simulink model "pidcontrol_withmotor"  (Simulink 7.1)
settings: Solver=ode45  StartTime=0.0  StopTime=10  RelTol=1e-3
values from neighbouring files (symbols this model uses):
  f0 = 7.847    [pid_parameters.m]
  f1 = -25.831    [pid_parameters.m]
  g = 9.81    [pid_parameters.m]
  I = 0.00017701    [pid_parameters.m]
  Kd = 0.06*100    (= 6)    [pid_parameters.m]
  Ki = 0.028*100    (= 2.8)    [pid_parameters.m]
  Kp = 0.037*100    (= 3.7)    [pid_parameters.m]
  l = 0.14875    [pid_parameters.m]
  M = 0.703    [pid_parameters.m]
  m = 0.024    [pid_parameters.m]
settings Model: Creator=minakata  LastModifiedBy=minakata

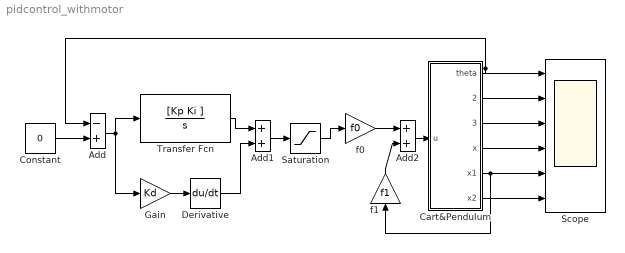
== system pidcontrol_withmotor ==
  Add : Sum  Inputs=-+  OutDataType=sfix(16)  OutScaling=2^-10
  Add1 : Sum  OutDataType=sfix(16)  OutScaling=2^-10
  Add2 : Sum  OutDataType=sfix(16)  OutScaling=2^-10
  Cart&Pendulum : Subsystem
  Constant : Constant  Value=0  OutDataType=sfix(16)  OutScaling=2^0
  Derivative : Derivative
  Gain : Gain  Gain=Kd  ParameterDataType=sfix(16)  ParameterScaling=2^0  OutDataType=sfix(16)  OutScaling=2^0
  Saturation : Saturate  UpperLimit=1  LowerLimit=-1  ZeroCross=off  OutDataType=sfix(16)  OutScaling=2^0
  Scope : Scope  NumInputPorts=6
      settings: TimeRange=10  YMin=0.095~-4.5e-007~-10~2e-015~2.5e-007~-15  YMax=0.105~-2e-007~12.5~1.3e-014~6e-007~15
  Transfer Fcn : TransferFcn  Numerator=[Kp Ki ]  Denominator=[ 1 0]
  f0 : Gain  Gain=f0  ParameterDataType=sfix(16)  ParameterScaling=2^0  OutDataType=sfix(16)  OutScaling=2^0
  f1 : Gain  Orientation=up  Gain=f1  ParameterDataType=sfix(16)  ParameterScaling=2^0  OutDataType=sfix(16)  OutScaling=2^0
  wires:
  Constant/1 -> Add/2
  Cart&Pendulum/1(theta) -> Add/1, Scope/1
  Add/1 -> Transfer Fcn/1, Gain/1
  Cart&Pendulum/2(theta1) -> Scope/2
  Cart&Pendulum/3(theta2) -> Scope/3
  Cart&Pendulum/4(x) -> Scope/4
  Cart&Pendulum/5(x1) -> Scope/5, f1/1
  Cart&Pendulum/6(x2) -> Scope/6
  Gain/1 -> Derivative/1
  Add1/1 -> Saturation/1
  Transfer Fcn/1 -> Add1/1
  Derivative/1 -> Add1/2
  Add2/1 -> Cart&Pendulum/1(u)
  f1/1 -> Add2/2
  f0/1 -> Add2/1
  Saturation/1 -> f0/1

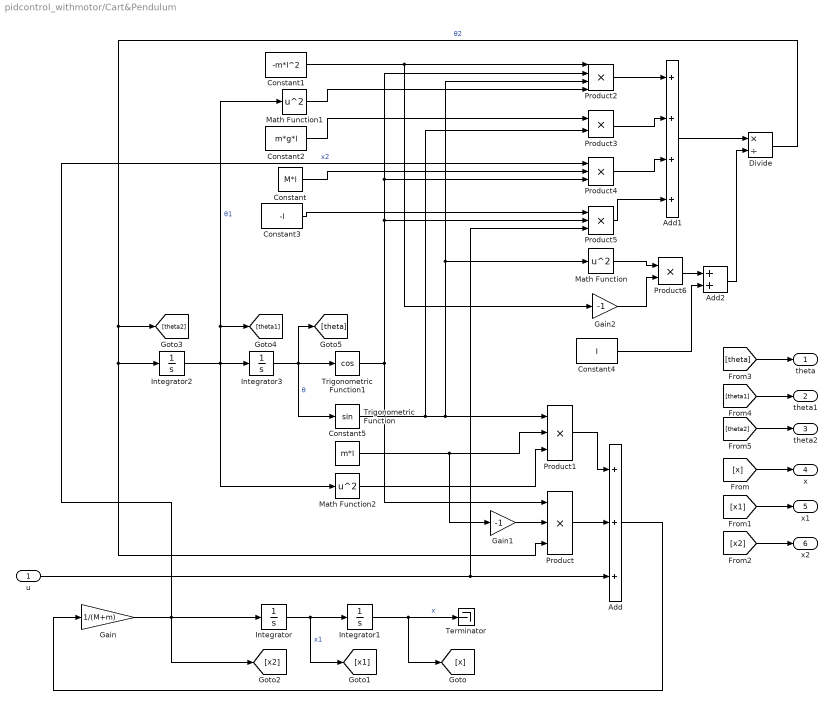
== system pidcontrol_withmotor/Cart&Pendulum ==
  u : Inport  OutDataType=sfix(16)  OutScaling=2^0
  Add : Sum  Inputs=+++  OutDataType=sfix(16)  OutScaling=2^-10
  Add1 : Sum  Inputs=++++  OutDataType=sfix(16)  OutScaling=2^-10
  Add2 : Sum  OutDataType=sfix(16)  OutScaling=2^-10
  Constant : Constant  Value=M*l  OutDataType=sfix(16)  OutScaling=2^0
  Constant1 : Constant  Value=-m*l^2  OutDataType=sfix(16)  OutScaling=2^0
  Constant2 : Constant  Value=m*g*l  OutDataType=sfix(16)  OutScaling=2^0
  Constant3 : Constant  Value=-l  OutDataType=sfix(16)  OutScaling=2^0
  Constant4 : Constant  Value=I  OutDataType=sfix(16)  OutScaling=2^0
  Constant5 : Constant  Value=m*l  OutDataType=sfix(16)  OutScaling=2^0
  Divide : Product  Inputs=*/  OutDataType=sfix(16)  OutScaling=2^-10
  Gain : Gain  Gain=1/(M+m)  ParameterDataType=sfix(16)  ParameterScaling=2^0  OutDataType=sfix(16)  OutScaling=2^0
  Gain1 : Gain  Gain=-1  ParameterDataType=sfix(16)  ParameterScaling=2^0  OutDataType=sfix(16)  OutScaling=2^0
  Gain2 : Gain  Gain=-1  ParameterDataType=sfix(16)  ParameterScaling=2^0  OutDataType=sfix(16)  OutScaling=2^0
  Integrator : Integrator
  Integrator1 : Integrator
  Integrator2 : Integrator
  Integrator3 : Integrator  InitialCondition=0.1
  Math Function : Math  Operator=square  OutDataType=sfix(16)  OutScaling=2^0  SaturateOnIntegerOverflow=on
  Math Function1 : Math  Operator=square  OutDataType=sfix(16)  OutScaling=2^0  SaturateOnIntegerOverflow=on
  Math Function2 : Math  Operator=square  OutDataType=sfix(16)  OutScaling=2^0  SaturateOnIntegerOverflow=on
  Product{,1,4..5} (4 alike) : Product  Inputs=3  OutDataType=sfix(16)  OutScaling=2^0  RndMeth=Zero
  Product2 : Product  Inputs=4  OutDataType=sfix(16)  OutScaling=2^0  RndMeth=Zero
  Product3 : Product  OutDataType=sfix(16)  OutScaling=2^0  RndMeth=Zero
  Product6 : Product  OutDataType=sfix(16)  OutScaling=2^0  RndMeth=Zero
  Terminator : Terminator
  Trigonometric Function : Trigonometry
  Trigonometric Function1 : Trigonometry  Operator=cos
  theta : Outport  OutDataType=sfix(16)  OutScaling=2^0
  theta1 : Outport  Port=2  OutDataType=sfix(16)  OutScaling=2^0
  theta2 : Outport  Port=3  OutDataType=sfix(16)  OutScaling=2^0
  x : Outport  Port=4  OutDataType=sfix(16)  OutScaling=2^0
  x1 : Outport  Port=5  OutDataType=sfix(16)  OutScaling=2^0
  x2 : Outport  Port=6  OutDataType=sfix(16)  OutScaling=2^0
  wires:
  [x] -> x/1
  [x1] -> x1/1
  [x2] -> x2/1
  [theta] -> theta/1
  [theta1] -> theta1/1
  [theta2] -> theta2/1
  Integrator1/1 -> Terminator/1, [x]  "x"
  Add/1 -> Gain/1
  u/1 -> Product5/3, Add/3
  Add1/1 -> Divide/1
  Add2/1 -> Divide/2
  Constant4/1 -> Add2/2
  Product6/1 -> Add2/1
  Math Function/1 -> Product6/1
  Product5/1 -> Add1/4
  Product4/1 -> Add1/3
  Product3/1 -> Add1/2
  Product2/1 -> Add1/1
  Constant3/1 -> Product5/1
  Constant2/1 -> Product3/1
  Constant1/1 -> Product2/1, Gain2/1
  Product1/1 -> Add/1
  Trigonometric Function1/1 -> Product2/2, Product4/3, Product5/2, Product/1
  Product/1 -> Add/2
  Constant/1 -> Product4/2
  Trigonometric Function/1 -> Product3/2, Product2/3, Math Function/1, Product1/1
  Integrator3/1 -> Trigonometric Function/1, Trigonometric Function1/1, [theta]  "θ"
  Integrator2/1 -> [theta1], Math Function1/1, Integrator3/1, Math Function2/1  "θ1"
  Divide/1 -> Integrator2/1, Product/3, [theta2]  "θ2"
  Integrator/1 -> Integrator1/1, [x1]  "x1"
  Gain/1 -> Product4/1, Integrator/1, [x2]  "x2"
  Math Function1/1 -> Product2/4
  Gain2/1 -> Product6/2
  Gain1/1 -> Product/2
  Math Function2/1 -> Product1/3
  Constant5/1 -> Product1/2, Gain1/1
